simulink model "Practica6simulink"  (R2024b)
settings: Solver=VariableStepAuto  StartTime=0.0  StopTime=0.010  RelTol=1e-3
values from neighbouring files (symbols this model uses):
  C = 10e-6    (= 1e-05)    [Practica6.m]
  L = 2e-3    (= 0.002)    [Practica6.m]
  R = 10    [Practica6.m]
  Uin = 32    [Practica6.m]    (also in Practica7ODE (1).m = 5)

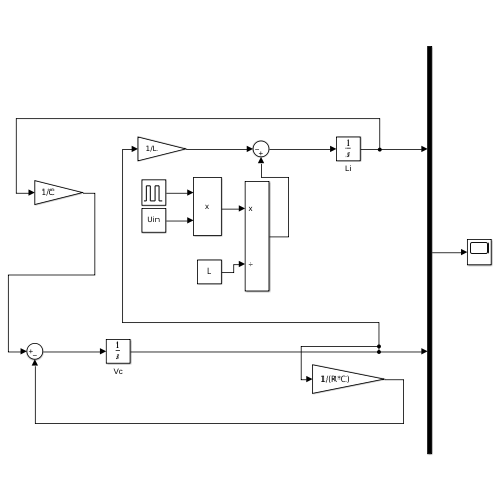
[thumbnail: Simulink's stored preview of the top-level diagram]
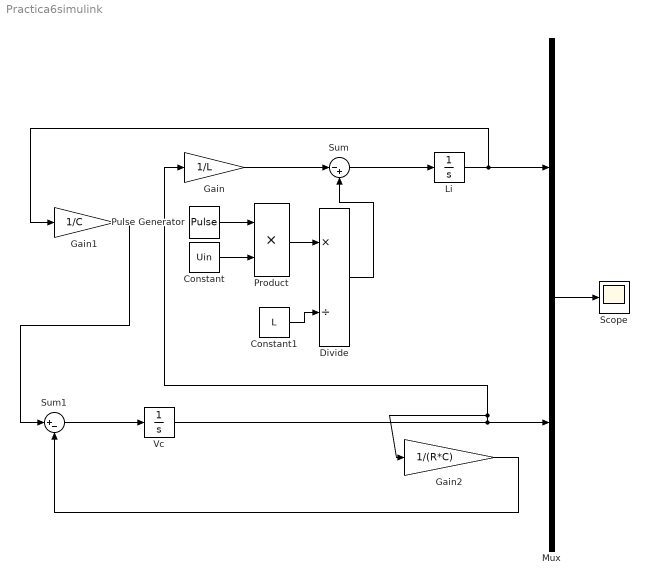
== system Practica6simulink ==
  Constant : Constant  Value=Uin
  Constant1 : Constant  Value=L
  Divide : Product  Inputs=*/
  Gain : Gain  Gain=1/L
  Gain1 : Gain  Gain=1/C
  Gain2 : Gain  Gain=1/(R*C)
  Li : Integrator
  Mux : Mux  Inputs=2
  Product : Product
  Pulse Generator : DiscretePulseGenerator  PulseType=Time based  Period=1/100e3  PulseWidth=40
  Scope : Scope
  Sum : Sum  Inputs=|-+
  Sum1 : Sum  Inputs=|+-
  Vc : Integrator
  wires:
  Constant/1 -> Product/2
  Product/1 -> Divide/1
  Constant1/1 -> Divide/2
  Gain/1 -> Sum/1
  Divide/1 -> Sum/2
  Sum/1 -> Li/1
  Li/1 -> Gain1/1, Mux/1
  Mux/1 -> Scope/1
  Gain1/1 -> Sum1/1
  Gain2/1 -> Sum1/2
  Sum1/1 -> Vc/1
  Vc/1 -> Gain2/1, Gain/1, Mux/2
  Pulse Generator/1 -> Product/1
